simulink model "Linear_Plant_LQR"  (R2024b)
settings: Solver=VariableStepAuto  StartTime=0.0  StopTime=300  RelTol=1e-3
settings Model: Creator=aryaman  LastModifiedBy=aryaman
settings DataIOCC: SaveFormat=StructureWithTime

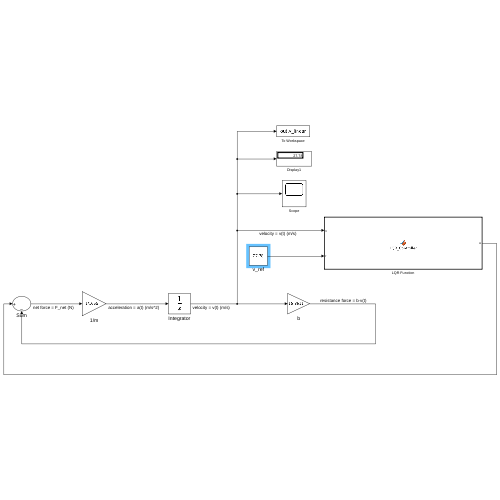
[thumbnail: Simulink's stored preview of the top-level diagram]
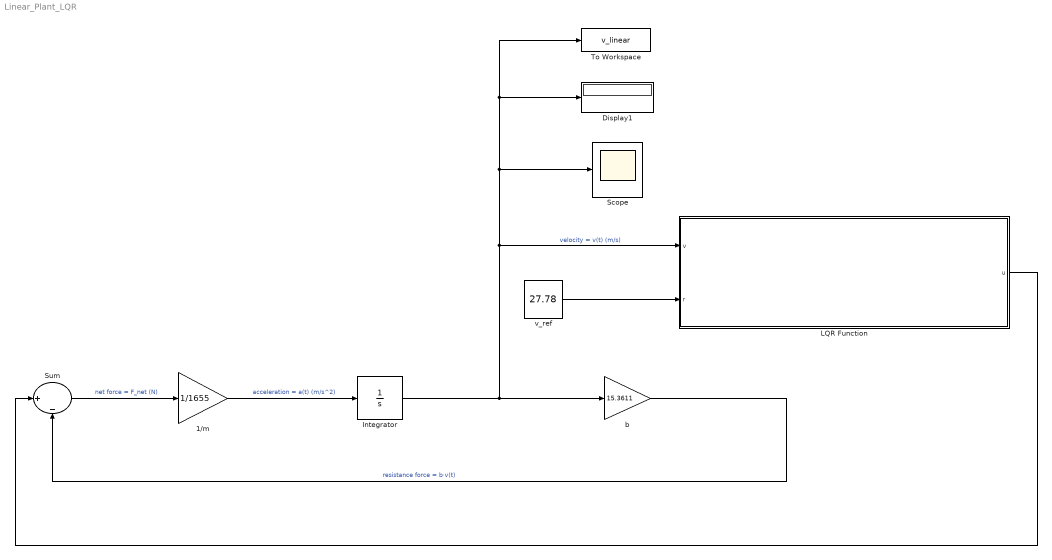
== system Linear_Plant_LQR ==
  1/m : Gain  Gain=1/1655
  Display1 : Display
  Integrator : Integrator
  LQR Function : MATLAB Function  TreatAsAtomicUnit=on
  Scope : Scope
  Sum : Sum  Inputs=||+|-
  To Workspace : ToWorkspace  VariableName=v_linear  SampleTime=-1
  b : Gain  Gain=15.3611
  v_ref : Constant  Value=27.78
  wires:
  Sum/1 -> 1/m/1  "net force = F_net (N)"
  1/m/1 -> Integrator/1  "acceleration = a(t) (m/s^2)"
  Integrator/1 -> b/1, To Workspace/1, Display1/1, Scope/1, LQR Function/1(v)  "velocity = v(t) (m/s)"
  b/1 -> Sum/2  "resistance force = b·v(t)"
  v_ref/1 -> LQR Function/2(r)
  LQR Function/1(u) -> Sum/1

== matlab function Linear_Plant_LQR/LQR Function ==
  data: v input; u output; r input
function u = LQR_Controller(v, r)
K = 33.9944;
Nbar = 49.3555;

u = -K * v + Nbar * r;
end
